simulink library "Cooling"  (R2024a)
settings: Solver=VariableStepAuto  StartTime=0.0  StopTime=10.0  RelTol=1e-3
values from neighbouring files (symbols this model uses):
  VehicleState : value not decoded    [StateMachine.sldd]
undefined symbols (not defined in the file or in its folder): raptor_xcp_function
libraries: $bdroot x11, Raptor_lib x9, simulink x6, Utilities x3
settings Model: Creator=serga  LastModifiedBy=hyuga
settings ConfigComp: CovBoundaryAbsTol=1.0e-5

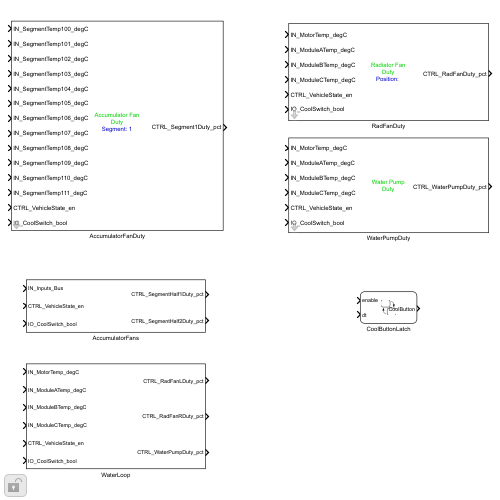
[thumbnail: Simulink's stored preview of the top-level diagram]
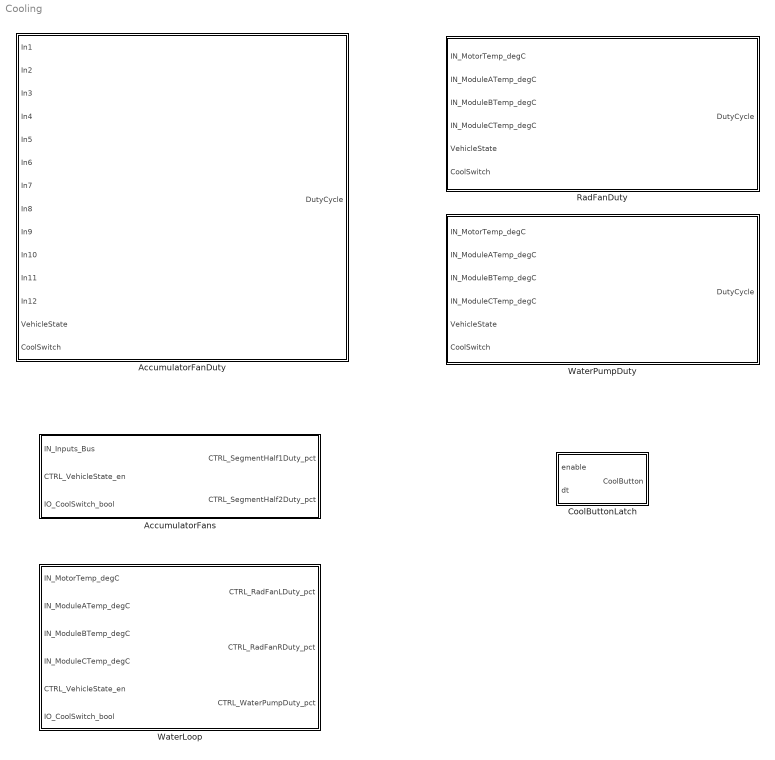
== system Cooling ==
  AccumulatorFanDuty : Subsystem  mask{pos='1'}
      mask prompts: pos "Segment"
      mask Display:
      | color('green')
      | disp('Accumulator Fan\nDuty\n\n');
      | color('blue')
      | disp(['\nSegment: ' pos]);
      | color('black')
      | port_label('input', 1, ['IN_SegmentTemp' pos '00_degC']);
      | port_label('input', 2, ['IN_SegmentTemp' pos '01_degC']);
      | port_label('input', 3, ['IN_SegmentTemp' pos '02_degC']);
      | port_label('input', 4, ['IN_SegmentTemp' pos '03_degC']);
      | port_label('input', 5, ['IN_SegmentTemp' pos '04_degC']);
      | port_label('input', 6, ['IN_SegmentTemp' pos '05_degC']);
      | port_label('input', 7, ['IN_SegmentTemp' pos '06_degC']);
      | port_label('input', 8, ['IN_SegmentTemp' pos '07_degC']);
      | port_label('input', 9, ['IN_SegmentTemp' pos '08_degC']);
      | port_label('input', 10, ['IN_SegmentTemp' pos '09_degC']);
      | port_label('input', 11, ['IN_SegmentTemp' pos '10_degC']);
      | port_label('input', 12, ['IN_SegmentTemp' pos '11_degC']);
      | port_label('input', 13, 'CTRL_VehicleState_en');
      | port_label('input', 14, 'IO_CoolSwitch_bool');
      | port_label('output', 1, ['CTRL_Segment' pos 'Duty_pct']);
  AccumulatorFans : Subsystem
  CoolButtonLatch : Stateflow chart  TreatAsAtomicUnit=on
  RadFanDuty : Subsystem  mask{pos=''}
      mask prompts: pos "Position"
      mask Display:
      | color('green')
      | disp('Radiator Fan\nDuty\n');
      | color('blue')
      | disp(['\n\nPosition: ' pos]);
      | color('black')
      | port_label('input', 1, 'IN_MotorTemp_degC');
      | port_label('input', 2, 'IN_ModuleATemp_degC');
      | port_label('input', 3, 'IN_ModuleBTemp_degC');
      | port_label('input', 4, 'IN_ModuleCTemp_degC');
      | port_label('input', 5, 'CTRL_VehicleState_en');
      | port_label('input', 6, 'IO_CoolSwitch_bool');
      | port_label('output', 1, ['CTRL_RadFan' pos 'Duty_pct']);
  WaterLoop : Subsystem
  WaterPumpDuty : Subsystem
      mask Display:
      | color('green')
      | disp('Water Pump\nDuty');
      | % color('blue')
      | % disp(['\nPosition: ' pos]);
      | color('black')
      | port_label('input', 1, 'IN_MotorTemp_degC');
      | port_label('input', 2, 'IN_ModuleATemp_degC');
      | port_label('input', 3, 'IN_ModuleBTemp_degC');
      | port_label('input', 4, 'IN_ModuleCTemp_degC');
      | port_label('input', 5, 'CTRL_VehicleState_en');
      | port_label('input', 6, 'IO_CoolSwitch_bool');
      | port_label('output', 1, 'CTRL_WaterPumpDuty_pct');

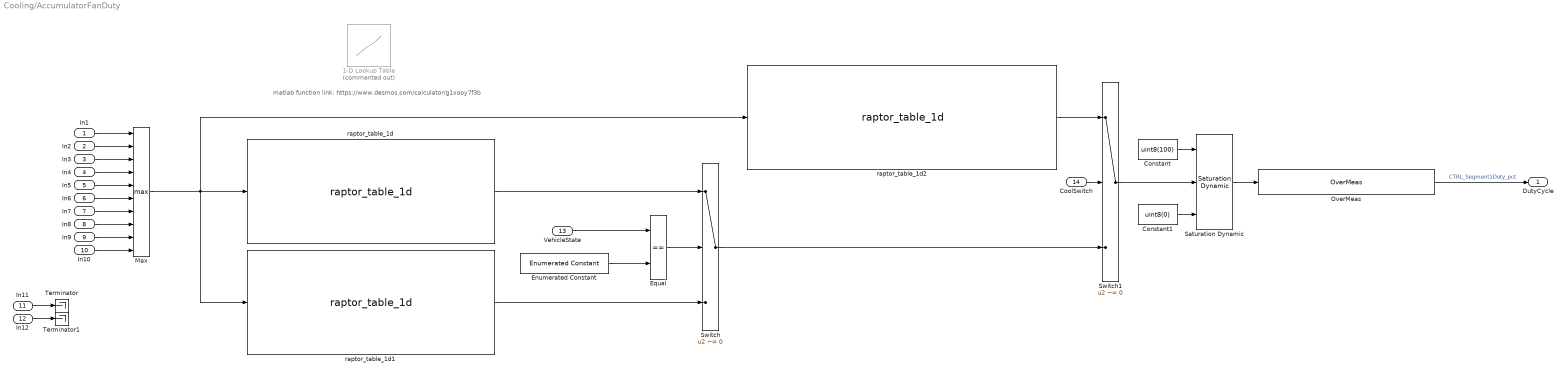
== system Cooling/AccumulatorFanDuty ==
  note: matlab function link: https://www.desmos.com/calculator/g1xooy7f3b
  In1 : Inport
  In2 : Inport  Port=2
  In3 : Inport  Port=3
  In4 : Inport  Port=4
  In5 : Inport  Port=5
  In6 : Inport  Port=6
  In7 : Inport  Port=7
  In8 : Inport  Port=8
  In9 : Inport  Port=9
  In10 : Inport  Port=10
  In11 : Inport  Port=11
  In12 : Inport  Port=12
  VehicleState : Inport  Port=13
  CoolSwitch : Inport  Port=14
  1-D Lookup Table : Lookup_n-D  Commented=on  NumberOfTableDimensions=1  BreakpointsForDimension1=[0:100]  Table=min(((tanh(([0:100]-40)/20)*50+50).^1.03),100)  InternalRulePriority=Speed  RndMeth=Simplest
  Constant : Constant  Value=uint8(100)
  Constant1 : Constant  Value=uint8(0)
  Enumerated Constant : simulink/Sources/Enumerated Constant  OutDataTypeStr=Enum: VehicleState  Value=VehicleState.ReadyToMove  SampleTime=inf
  Equal : RelationalOperator  Operator===  OutDataTypeStr=boolean  RndMeth=Simplest  InputSameDT=off
  Max : MinMax  Function=max  Inputs=10
  OverMeas : Utilities/OverMeas  sigName=['CTRL_Segment' pos 'Duty_pct']  minimum=0  maximum=100
  Saturation Dynamic : simulink/Discontinuities/Saturation Dynamic  OutMin=[]  OutMax=[]  OutDataTypeStr=Inherit: Same as second input  OutDataType=fixdt(1, 16)  OutScaling=2^-10  DoSatur=off
  Switch : Switch  Criteria=u2 ~= 0  SaturateOnIntegerOverflow=off  InputSameDT=off
  Switch1 : Switch  Criteria=u2 ~= 0  SaturateOnIntegerOverflow=off  InputSameDT=off
  Terminator : Terminator
  Terminator1 : Terminator
  raptor_table_1d : Raptor_lib/Table Lookup/raptor_table_1d  dataName=['CTRL_Segment' pos 'TempToHVDutyCycle']  initValue=min(((tanh(([0:100]-40)/20)*50+50).^1.03),80)  dataType=single  storage=Calibration  initValueX=[0:100]  dataTypeXY=single  storageXY=Calibration  calVisible=on  showTable=on  calGain=1.0  calOffset=0.0  calMax=Inf  calMin=-Inf  calFormat='-1'  calUnit='pct'  calHelp=''  showBreakpoint=on  dataNameX=[]  calGainX=1.0  calOffsetX=0.0  calMaxX=Inf  calMinX=-Inf  calFormatX='-1'  calUnitX='degC'  calHelpX=''  calAccess=1  calFunction=raptor_xcp_function(gcb)  measureEnable=off  mName=['Data1D_Output']
      settings: SourceProductName=Raptor
  raptor_table_1d1 : Raptor_lib/Table Lookup/raptor_table_1d  dataName=['CTRL_Segment' pos 'TempToLVDutyCycle']  initValue=min(((tanh(([0:100]-50)/20)*50+50).^1.03),50)  dataType=single  storage=Calibration  initValueX=[0:100]  dataTypeXY=single  storageXY=Calibration  calVisible=on  showTable=on  calGain=1.0  calOffset=0.0  calMax=Inf  calMin=-Inf  calFormat='-1'  calUnit='pct'  calHelp=''  showBreakpoint=on  dataNameX=[]  calGainX=1.0  calOffsetX=0.0  calMaxX=Inf  calMinX=-Inf  calFormatX='-1'  calUnitX='degC'  calHelpX=''  calAccess=1  calFunction=raptor_xcp_function(gcb)  measureEnable=off  mName=['Data1D_Output']
      settings: SourceProductName=Raptor
  raptor_table_1d2 : Raptor_lib/Table Lookup/raptor_table_1d  dataName=['CTRL_Segment' pos 'TempToDutyCycleOverride']  initValue=min(((tanh(([0:100]-25)/20)*50+50).^1.03),100)  dataType=single  storage=Calibration  initValueX=[0:100]  dataTypeXY=single  storageXY=Calibration  calVisible=on  showTable=on  calGain=1.0  calOffset=0.0  calMax=Inf  calMin=-Inf  calFormat='-1'  calUnit='pct'  calHelp=''  showBreakpoint=on  dataNameX=[]  calGainX=1.0  calOffsetX=0.0  calMaxX=Inf  calMinX=-Inf  calFormatX='-1'  calUnitX='degC'  calHelpX=''  calAccess=1  calFunction=raptor_xcp_function(gcb)  measureEnable=off  mName=['Data1D_Output']
      settings: SourceProductName=Raptor
  DutyCycle : Outport
  wires:
  In1/1 -> Max/1
  In2/1 -> Max/2
  In3/1 -> Max/3
  In4/1 -> Max/4
  In5/1 -> Max/5
  In6/1 -> Max/6
  In7/1 -> Max/7
  In8/1 -> Max/8
  In9/1 -> Max/9
  In10/1 -> Max/10
  In11/1 -> Terminator/1
  In12/1 -> Terminator1/1
  Max/1 -> raptor_table_1d1/1, raptor_table_1d2/1, raptor_table_1d/1
  raptor_table_1d/1 -> Switch/1
  VehicleState/1 -> Equal/1
  Enumerated Constant/1 -> Equal/2
  Equal/1 -> Switch/2
  Switch/1 -> Switch1/3
  raptor_table_1d1/1 -> Switch/3
  CoolSwitch/1 -> Switch1/2
  raptor_table_1d2/1 -> Switch1/1
  Switch1/1 -> Saturation Dynamic/2
  Constant/1 -> Saturation Dynamic/1
  Constant1/1 -> Saturation Dynamic/3
  Saturation Dynamic/1 -> OverMeas/1
  OverMeas/1 -> DutyCycle/1  "CTRL_Segment1Duty_pct"

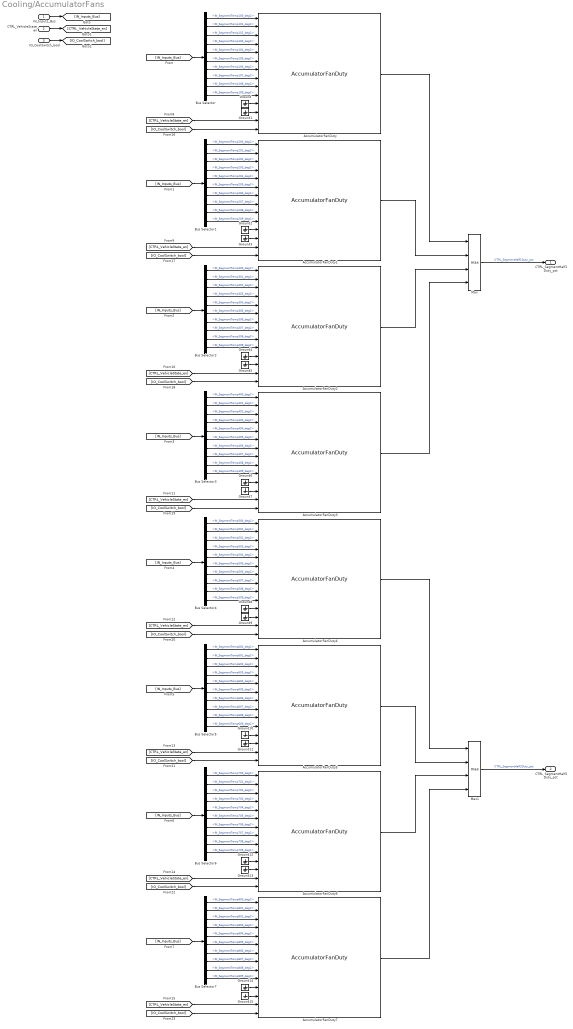
== system Cooling/AccumulatorFans ==
  IN_Inputs_Bus : Inport
  CTRL_VehicleState_en : Inport  Port=2
  IO_CoolSwitch_bool : Inport  Port=3
  AccumulatorFanDuty : $bdroot/AccumulatorFanDuty  pos='1'
  AccumulatorFanDuty1 : $bdroot/AccumulatorFanDuty  pos='2'
  AccumulatorFanDuty2 : $bdroot/AccumulatorFanDuty  pos='3'
  AccumulatorFanDuty3 : $bdroot/AccumulatorFanDuty  pos='4'
  AccumulatorFanDuty4 : $bdroot/AccumulatorFanDuty  pos='5'
  AccumulatorFanDuty5 : $bdroot/AccumulatorFanDuty  pos='6'
  AccumulatorFanDuty6 : $bdroot/AccumulatorFanDuty  pos='7'
  AccumulatorFanDuty7 : $bdroot/AccumulatorFanDuty  pos='8'
  Bus Selector : BusSelector  OutputSignals=IN_STMM_Bus.IN_Segment1Temp_Bus.IN_SegmentTemp100_degC,IN_STMM_Bus.IN_Segment1Temp_Bus.IN_SegmentTemp101_degC,IN_STMM_Bus.IN_Segment1Temp_Bus.IN_SegmentTemp102_degC,IN_STMM_Bus.IN_Segment1Temp_Bus.IN_SegmentTemp103_degC,IN_STMM_Bus.IN_Segment1Temp_Bus.IN_SegmentTemp104_degC,IN_STMM_Bus.IN_Segment1Temp_Bus.IN_SegmentTemp105_degC,IN_STMM_Bus.IN_Segment1Temp_Bus.IN_SegmentTemp106_degC,IN_STMM_Bus.IN_Segment1Temp_Bus.IN_SegmentTemp107_degC,IN_STMM_Bus.IN_Segment1Temp_Bus.IN_SegmentTemp108_degC,IN_STMM_Bus.IN_Segment1Temp_Bus.IN_SegmentTemp109_degC
  Bus Selector1 : BusSelector  OutputSignals=IN_STMM_Bus.IN_Segment2Temp_Bus.IN_SegmentTemp200_degC,IN_STMM_Bus.IN_Segment2Temp_Bus.IN_SegmentTemp201_degC,IN_STMM_Bus.IN_Segment2Temp_Bus.IN_SegmentTemp202_degC,IN_STMM_Bus.IN_Segment2Temp_Bus.IN_SegmentTemp203_degC,IN_STMM_Bus.IN_Segment2Temp_Bus.IN_SegmentTemp204_degC,IN_STMM_Bus.IN_Segment2Temp_Bus.IN_SegmentTemp205_degC,IN_STMM_Bus.IN_Segment2Temp_Bus.IN_SegmentTemp206_degC,IN_STMM_Bus.IN_Segment2Temp_Bus.IN_SegmentTemp207_degC,IN_STMM_Bus.IN_Segment2Temp_Bus.IN_SegmentTemp208_degC,IN_STMM_Bus.IN_Segment2Temp_Bus.IN_SegmentTemp209_degC
  Bus Selector2 : BusSelector  OutputSignals=IN_STMM_Bus.IN_Segment3Temp_Bus.IN_SegmentTemp300_degC,IN_STMM_Bus.IN_Segment3Temp_Bus.IN_SegmentTemp301_degC,IN_STMM_Bus.IN_Segment3Temp_Bus.IN_SegmentTemp302_degC,IN_STMM_Bus.IN_Segment3Temp_Bus.IN_SegmentTemp303_degC,IN_STMM_Bus.IN_Segment3Temp_Bus.IN_SegmentTemp304_degC,IN_STMM_Bus.IN_Segment3Temp_Bus.IN_SegmentTemp305_degC,IN_STMM_Bus.IN_Segment3Temp_Bus.IN_SegmentTemp306_degC,IN_STMM_Bus.IN_Segment3Temp_Bus.IN_SegmentTemp307_degC,IN_STMM_Bus.IN_Segment3Temp_Bus.IN_SegmentTemp308_degC,IN_STMM_Bus.IN_Segment3Temp_Bus.IN_SegmentTemp309_degC
  Bus Selector3 : BusSelector  OutputSignals=IN_STMM_Bus.IN_Segment4Temp_Bus.IN_SegmentTemp400_degC,IN_STMM_Bus.IN_Segment4Temp_Bus.IN_SegmentTemp401_degC,IN_STMM_Bus.IN_Segment4Temp_Bus.IN_SegmentTemp402_degC,IN_STMM_Bus.IN_Segment4Temp_Bus.IN_SegmentTemp403_degC,IN_STMM_Bus.IN_Segment4Temp_Bus.IN_SegmentTemp404_degC,IN_STMM_Bus.IN_Segment4Temp_Bus.IN_SegmentTemp405_degC,IN_STMM_Bus.IN_Segment4Temp_Bus.IN_SegmentTemp406_degC,IN_STMM_Bus.IN_Segment4Temp_Bus.IN_SegmentTemp407_degC,IN_STMM_Bus.IN_Segment4Temp_Bus.IN_SegmentTemp408_degC,IN_STMM_Bus.IN_Segment4Temp_Bus.IN_SegmentTemp409_degC
  Bus Selector4 : BusSelector  OutputSignals=IN_STMM_Bus.IN_Segment5Temp_Bus.IN_SegmentTemp500_degC,IN_STMM_Bus.IN_Segment5Temp_Bus.IN_SegmentTemp501_degC,IN_STMM_Bus.IN_Segment5Temp_Bus.IN_SegmentTemp502_degC,IN_STMM_Bus.IN_Segment5Temp_Bus.IN_SegmentTemp503_degC,IN_STMM_Bus.IN_Segment5Temp_Bus.IN_SegmentTemp504_degC,IN_STMM_Bus.IN_Segment5Temp_Bus.IN_SegmentTemp505_degC,IN_STMM_Bus.IN_Segment5Temp_Bus.IN_SegmentTemp506_degC,IN_STMM_Bus.IN_Segment5Temp_Bus.IN_SegmentTemp507_degC,IN_STMM_Bus.IN_Segment5Temp_Bus.IN_SegmentTemp508_degC,IN_STMM_Bus.IN_Segment5Temp_Bus.IN_SegmentTemp509_degC
  Bus Selector5 : BusSelector  OutputSignals=IN_STMM_Bus.IN_Segment6Temp_Bus.IN_SegmentTemp600_degC,IN_STMM_Bus.IN_Segment6Temp_Bus.IN_SegmentTemp601_degC,IN_STMM_Bus.IN_Segment6Temp_Bus.IN_SegmentTemp602_degC,IN_STMM_Bus.IN_Segment6Temp_Bus.IN_SegmentTemp603_degC,IN_STMM_Bus.IN_Segment6Temp_Bus.IN_SegmentTemp604_degC,IN_STMM_Bus.IN_Segment6Temp_Bus.IN_SegmentTemp605_degC,IN_STMM_Bus.IN_Segment6Temp_Bus.IN_SegmentTemp606_degC,IN_STMM_Bus.IN_Segment6Temp_Bus.IN_SegmentTemp607_degC,IN_STMM_Bus.IN_Segment6Temp_Bus.IN_SegmentTemp608_degC,IN_STMM_Bus.IN_Segment6Temp_Bus.IN_SegmentTemp609_degC
  Bus Selector6 : BusSelector  OutputSignals=IN_STMM_Bus.IN_Segment7Temp_Bus.IN_SegmentTemp700_degC,IN_STMM_Bus.IN_Segment7Temp_Bus.IN_SegmentTemp701_degC,IN_STMM_Bus.IN_Segment7Temp_Bus.IN_SegmentTemp702_degC,IN_STMM_Bus.IN_Segment7Temp_Bus.IN_SegmentTemp703_degC,IN_STMM_Bus.IN_Segment7Temp_Bus.IN_SegmentTemp704_degC,IN_STMM_Bus.IN_Segment7Temp_Bus.IN_SegmentTemp705_degC,IN_STMM_Bus.IN_Segment7Temp_Bus.IN_SegmentTemp706_degC,IN_STMM_Bus.IN_Segment7Temp_Bus.IN_SegmentTemp707_degC,IN_STMM_Bus.IN_Segment7Temp_Bus.IN_SegmentTemp708_degC,IN_STMM_Bus.IN_Segment7Temp_Bus.IN_SegmentTemp709_degC
  Bus Selector7 : BusSelector  OutputSignals=IN_STMM_Bus.IN_Segment8Temp_Bus.IN_SegmentTemp800_degC,IN_STMM_Bus.IN_Segment8Temp_Bus.IN_SegmentTemp801_degC,IN_STMM_Bus.IN_Segment8Temp_Bus.IN_SegmentTemp802_degC,IN_STMM_Bus.IN_Segment8Temp_Bus.IN_SegmentTemp803_degC,IN_STMM_Bus.IN_Segment8Temp_Bus.IN_SegmentTemp804_degC,IN_STMM_Bus.IN_Segment8Temp_Bus.IN_SegmentTemp805_degC,IN_STMM_Bus.IN_Segment8Temp_Bus.IN_SegmentTemp806_degC,IN_STMM_Bus.IN_Segment8Temp_Bus.IN_SegmentTemp807_degC,IN_STMM_Bus.IN_Segment8Temp_Bus.IN_SegmentTemp808_degC,IN_STMM_Bus.IN_Segment8Temp_Bus.IN_SegmentTemp809_degC
  Ground{,1..15} (16 alike) : Ground
  Max : MinMax  Function=max  Inputs=4
  Max1 : MinMax  Function=max  Inputs=4
  CTRL_SegmentHalf1Duty_pct : Outport
  CTRL_SegmentHalf2Duty_pct : Outport  Port=2
  wires:
  Max1/1 -> CTRL_SegmentHalf2Duty_pct/1  "CTRL_SegmentHalf2Duty_pct"
  AccumulatorFanDuty7/1 -> Max1/4
  AccumulatorFanDuty6/1 -> Max1/3
  AccumulatorFanDuty5/1 -> Max1/2
  AccumulatorFanDuty4/1 -> Max1/1
  Max/1 -> CTRL_SegmentHalf1Duty_pct/1  "CTRL_SegmentHalf1Duty_pct"
  AccumulatorFanDuty3/1 -> Max/4
  AccumulatorFanDuty2/1 -> Max/3
  AccumulatorFanDuty1/1 -> Max/2
  AccumulatorFanDuty/1 -> Max/1
  [IO_CoolSwitch_bool] -> AccumulatorFanDuty7/14
  [IO_CoolSwitch_bool] -> AccumulatorFanDuty6/14
  [IO_CoolSwitch_bool] -> AccumulatorFanDuty5/14
  [IO_CoolSwitch_bool] -> AccumulatorFanDuty4/14
  [IO_CoolSwitch_bool] -> AccumulatorFanDuty3/14
  [IO_CoolSwitch_bool] -> AccumulatorFanDuty2/14
  [IO_CoolSwitch_bool] -> AccumulatorFanDuty1/14
  [IO_CoolSwitch_bool] -> AccumulatorFanDuty/14
  [CTRL_VehicleState_en] -> AccumulatorFanDuty7/13
  [CTRL_VehicleState_en] -> AccumulatorFanDuty6/13
  [CTRL_VehicleState_en] -> AccumulatorFanDuty5/13
  [CTRL_VehicleState_en] -> AccumulatorFanDuty4/13
  [CTRL_VehicleState_en] -> AccumulatorFanDuty3/13
  [CTRL_VehicleState_en] -> AccumulatorFanDuty2/13
  [CTRL_VehicleState_en] -> AccumulatorFanDuty1/13
  [CTRL_VehicleState_en] -> AccumulatorFanDuty/13
  [IN_Inputs_Bus] -> Bus Selector7/1
  [IN_Inputs_Bus] -> Bus Selector6/1
  [IN_Inputs_Bus] -> Bus Selector5/1
  [IN_Inputs_Bus] -> Bus Selector4/1
  [IN_Inputs_Bus] -> Bus Selector3/1
  [IN_Inputs_Bus] -> Bus Selector2/1
  [IN_Inputs_Bus] -> Bus Selector1/1
  [IN_Inputs_Bus] -> Bus Selector/1
  IO_CoolSwitch_bool/1 -> [IO_CoolSwitch_bool]
  CTRL_VehicleState_en/1 -> [CTRL_VehicleState_en]
  IN_Inputs_Bus/1 -> [IN_Inputs_Bus]
  Bus Selector7/10 -> AccumulatorFanDuty7/10  "<IN_SegmentTemp809_degC>"
  Bus Selector7/9 -> AccumulatorFanDuty7/9  "<IN_SegmentTemp808_degC>"
  Bus Selector7/8 -> AccumulatorFanDuty7/8  "<IN_SegmentTemp807_degC>"
  Bus Selector7/7 -> AccumulatorFanDuty7/7  "<IN_SegmentTemp806_degC>"
  Bus Selector7/6 -> AccumulatorFanDuty7/6  "<IN_SegmentTemp805_degC>"
  Bus Selector7/5 -> AccumulatorFanDuty7/5  "<IN_SegmentTemp804_degC>"
  Bus Selector7/4 -> AccumulatorFanDuty7/4  "<IN_SegmentTemp803_degC>"
  Bus Selector7/3 -> AccumulatorFanDuty7/3  "<IN_SegmentTemp802_degC>"
  Bus Selector7/2 -> AccumulatorFanDuty7/2  "<IN_SegmentTemp801_degC>"
  Bus Selector7/1 -> AccumulatorFanDuty7/1  "<IN_SegmentTemp800_degC>"
  Bus Selector6/10 -> AccumulatorFanDuty6/10  "<IN_SegmentTemp709_degC>"
  Bus Selector6/9 -> AccumulatorFanDuty6/9  "<IN_SegmentTemp708_degC>"
  Bus Selector6/8 -> AccumulatorFanDuty6/8  "<IN_SegmentTemp707_degC>"
  Bus Selector6/7 -> AccumulatorFanDuty6/7  "<IN_SegmentTemp706_degC>"
  Bus Selector6/6 -> AccumulatorFanDuty6/6  "<IN_SegmentTemp705_degC>"
  Bus Selector6/5 -> AccumulatorFanDuty6/5  "<IN_SegmentTemp704_degC>"
  Bus Selector6/4 -> AccumulatorFanDuty6/4  "<IN_SegmentTemp703_degC>"
  Bus Selector6/3 -> AccumulatorFanDuty6/3  "<IN_SegmentTemp702_degC>"
  Bus Selector6/2 -> AccumulatorFanDuty6/2  "<IN_SegmentTemp701_degC>"
  Bus Selector6/1 -> AccumulatorFanDuty6/1  "<IN_SegmentTemp700_degC>"
  Bus Selector5/10 -> AccumulatorFanDuty5/10  "<IN_SegmentTemp609_degC>"
  Bus Selector5/9 -> AccumulatorFanDuty5/9  "<IN_SegmentTemp608_degC>"
  Bus Selector5/8 -> AccumulatorFanDuty5/8  "<IN_SegmentTemp607_degC>"
  Bus Selector5/7 -> AccumulatorFanDuty5/7  "<IN_SegmentTemp606_degC>"
  Bus Selector5/6 -> AccumulatorFanDuty5/6  "<IN_SegmentTemp605_degC>"
  Bus Selector5/5 -> AccumulatorFanDuty5/5  "<IN_SegmentTemp604_degC>"
  Bus Selector5/4 -> AccumulatorFanDuty5/4  "<IN_SegmentTemp603_degC>"
  Bus Selector5/3 -> AccumulatorFanDuty5/3  "<IN_SegmentTemp602_degC>"
  Bus Selector5/2 -> AccumulatorFanDuty5/2  "<IN_SegmentTemp601_degC>"
  Bus Selector5/1 -> AccumulatorFanDuty5/1  "<IN_SegmentTemp600_degC>"
  Bus Selector4/10 -> AccumulatorFanDuty4/10  "<IN_SegmentTemp509_degC>"
  Bus Selector4/9 -> AccumulatorFanDuty4/9  "<IN_SegmentTemp508_degC>"
  Bus Selector4/8 -> AccumulatorFanDuty4/8  "<IN_SegmentTemp507_degC>"
  Bus Selector4/7 -> AccumulatorFanDuty4/7  "<IN_SegmentTemp506_degC>"
  Bus Selector4/6 -> AccumulatorFanDuty4/6  "<IN_SegmentTemp505_degC>"
  Bus Selector4/5 -> AccumulatorFanDuty4/5  "<IN_SegmentTemp504_degC>"
  Bus Selector4/4 -> AccumulatorFanDuty4/4  "<IN_SegmentTemp503_degC>"
  Bus Selector4/3 -> AccumulatorFanDuty4/3  "<IN_SegmentTemp502_degC>"
  Bus Selector4/2 -> AccumulatorFanDuty4/2  "<IN_SegmentTemp501_degC>"
  Bus Selector4/1 -> AccumulatorFanDuty4/1  "<IN_SegmentTemp500_degC>"
  Bus Selector3/10 -> AccumulatorFanDuty3/10  "<IN_SegmentTemp409_degC>"
  Bus Selector3/9 -> AccumulatorFanDuty3/9  "<IN_SegmentTemp408_degC>"
  Bus Selector3/8 -> AccumulatorFanDuty3/8  "<IN_SegmentTemp407_degC>"
  Bus Selector3/7 -> AccumulatorFanDuty3/7  "<IN_SegmentTemp406_degC>"
  Bus Selector3/6 -> AccumulatorFanDuty3/6  "<IN_SegmentTemp405_degC>"
  Bus Selector3/5 -> AccumulatorFanDuty3/5  "<IN_SegmentTemp404_degC>"
  Bus Selector3/4 -> AccumulatorFanDuty3/4  "<IN_SegmentTemp403_degC>"
  Bus Selector3/3 -> AccumulatorFanDuty3/3  "<IN_SegmentTemp402_degC>"
  Bus Selector3/2 -> AccumulatorFanDuty3/2  "<IN_SegmentTemp401_degC>"
  Bus Selector3/1 -> AccumulatorFanDuty3/1  "<IN_SegmentTemp400_degC>"
  Bus Selector2/10 -> AccumulatorFanDuty2/10  "<IN_SegmentTemp309_degC>"
  Bus Selector2/9 -> AccumulatorFanDuty2/9  "<IN_SegmentTemp308_degC>"
  Bus Selector2/8 -> AccumulatorFanDuty2/8  "<IN_SegmentTemp307_degC>"
  Bus Selector2/7 -> AccumulatorFanDuty2/7  "<IN_SegmentTemp306_degC>"
  Bus Selector2/6 -> AccumulatorFanDuty2/6  "<IN_SegmentTemp305_degC>"
  Bus Selector2/5 -> AccumulatorFanDuty2/5  "<IN_SegmentTemp304_degC>"
  Bus Selector2/4 -> AccumulatorFanDuty2/4  "<IN_SegmentTemp303_degC>"
  Bus Selector2/3 -> AccumulatorFanDuty2/3  "<IN_SegmentTemp302_degC>"
  Bus Selector2/2 -> AccumulatorFanDuty2/2  "<IN_SegmentTemp301_degC>"
  Bus Selector2/1 -> AccumulatorFanDuty2/1  "<IN_SegmentTemp300_degC>"
  Bus Selector1/10 -> AccumulatorFanDuty1/10  "<IN_SegmentTemp209_degC>"
  Bus Selector1/9 -> AccumulatorFanDuty1/9  "<IN_SegmentTemp208_degC>"
  Bus Selector1/8 -> AccumulatorFanDuty1/8  "<IN_SegmentTemp207_degC>"
  Bus Selector1/7 -> AccumulatorFanDuty1/7  "<IN_SegmentTemp206_degC>"
  Bus Selector1/6 -> AccumulatorFanDuty1/6  "<IN_SegmentTemp205_degC>"
  Bus Selector1/5 -> AccumulatorFanDuty1/5  "<IN_SegmentTemp204_degC>"
  Bus Selector1/4 -> AccumulatorFanDuty1/4  "<IN_SegmentTemp203_degC>"
  Bus Selector1/3 -> AccumulatorFanDuty1/3  "<IN_SegmentTemp202_degC>"
  Bus Selector1/2 -> AccumulatorFanDuty1/2  "<IN_SegmentTemp201_degC>"
  Bus Selector1/1 -> AccumulatorFanDuty1/1  "<IN_SegmentTemp200_degC>"
  Bus Selector/10 -> AccumulatorFanDuty/10  "<IN_SegmentTemp109_degC>"
  Bus Selector/9 -> AccumulatorFanDuty/9  "<IN_SegmentTemp108_degC>"
  Bus Selector/8 -> AccumulatorFanDuty/8  "<IN_SegmentTemp107_degC>"
  Bus Selector/7 -> AccumulatorFanDuty/7  "<IN_SegmentTemp106_degC>"
  Bus Selector/6 -> AccumulatorFanDuty/6  "<IN_SegmentTemp105_degC>"
  Bus Selector/5 -> AccumulatorFanDuty/5  "<IN_SegmentTemp104_degC>"
  Bus Selector/4 -> AccumulatorFanDuty/4  "<IN_SegmentTemp103_degC>"
  Bus Selector/3 -> AccumulatorFanDuty/3  "<IN_SegmentTemp102_degC>"
  Bus Selector/2 -> AccumulatorFanDuty/2  "<IN_SegmentTemp101_degC>"
  Bus Selector/1 -> AccumulatorFanDuty/1  "<IN_SegmentTemp100_degC>"
  Ground/1 -> AccumulatorFanDuty/11
  Ground1/1 -> AccumulatorFanDuty/12
  Ground2/1 -> AccumulatorFanDuty1/11
  Ground3/1 -> AccumulatorFanDuty1/12
  Ground4/1 -> AccumulatorFanDuty2/11
  Ground5/1 -> AccumulatorFanDuty2/12
  Ground6/1 -> AccumulatorFanDuty3/11
  Ground7/1 -> AccumulatorFanDuty3/12
  Ground8/1 -> AccumulatorFanDuty4/11
  Ground9/1 -> AccumulatorFanDuty4/12
  Ground10/1 -> AccumulatorFanDuty5/11
  Ground11/1 -> AccumulatorFanDuty5/12
  Ground12/1 -> AccumulatorFanDuty6/11
  Ground13/1 -> AccumulatorFanDuty6/12
  Ground14/1 -> AccumulatorFanDuty7/11
  Ground15/1 -> AccumulatorFanDuty7/12

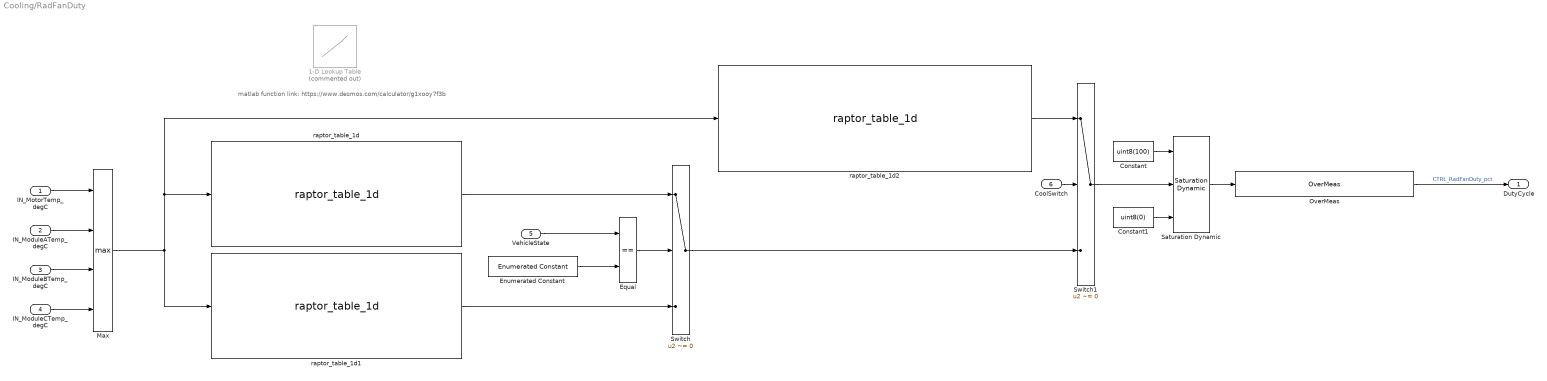
== system Cooling/RadFanDuty ==
  note: matlab function link: https://www.desmos.com/calculator/g1xooy7f3b
  IN_MotorTemp_degC : Inport
  IN_ModuleATemp_degC : Inport  Port=2
  IN_ModuleBTemp_degC : Inport  Port=3
  IN_ModuleCTemp_degC : Inport  Port=4
  VehicleState : Inport  Port=5
  CoolSwitch : Inport  Port=6
  1-D Lookup Table : Lookup_n-D  Commented=on  NumberOfTableDimensions=1  BreakpointsForDimension1=[0; 1; 2; 3; 4; 5; 6; 7; 8; 9; 10; 11; 12; 13; 14; 15; 16; 17; 18; 19; 20; 21; 22; 23; 24; 25; 26; 27; 28; 29; 30; 31; 32; 33; 34; 35; 36; 37; 38; 39; 40; 41; 42; 43; 44; 45; 46; 47; 48; 49; 50; 51; 52; 53; 54; 55; 56; 57; 58; 59; 60; 61; 62; 63; 64; 65; 66; 67; 68; 69; 70; 71; 72; 73; 74; 75; 76; 77; 78; 79; 80; 81; 82; 83; 84; 85; 86; 87; 88; 89; 90; 91; 92; 93; 94; 95; 96; 97; 98; 99; 100; 101; 102; 103; 104; 105; 106; 107; 108; 109; 110; 111; 112; 113; 114; 115; 116; 117; 118]  Table=[2, 2, 2, 2, 3, 3, 3, 4, 4, 5, 5, 5, 6, 7, 7, 8, 9, 10, 11, 12, 13, 14, 15, 17, 18, 20, 22, 23, 25, 28, 30, 32, 34, 37, 39, 42, 45, 48, 50, 53, 56, 59, 62, 65, 68, 70, 73, 76, 78, 81, 83, 85, 88, 90, 91, 93, 95, 97, 98, 99, 100, 100, 100, 100, 100, 100, 100, 100, 100, 100, 100, 100, 100, 100, 100, 100, 100, 100, 100, 100, 100, 100, 100, 100, 100, 100, 100, 100, 100, 100, 100, 100, 100, 100, 100, 100, 100, 100, 100, 100, 100, 100, 100, 100, 100, 100, 100, 100, 100, 100, 100, 100, 100, 100, 100, 100, 100, 100, 100]  InternalRulePriority=Speed  RndMeth=Simplest
  Constant : Constant  Value=uint8(100)
  Constant1 : Constant  Value=uint8(0)
  Enumerated Constant : simulink/Sources/Enumerated Constant  OutDataTypeStr=Enum: VehicleState  Value=VehicleState.ReadyToMove  SampleTime=inf
  Equal : RelationalOperator  Operator===  OutDataTypeStr=boolean  RndMeth=Simplest  InputSameDT=off
  Max : MinMax  Function=max  Inputs=4
  OverMeas : Utilities/OverMeas  sigName=['CTRL_RadFan' pos 'Duty_pct']  minimum=0  maximum=100
  Saturation Dynamic : simulink/Discontinuities/Saturation Dynamic  OutMin=[]  OutMax=[]  OutDataTypeStr=Inherit: Same as second input  OutDataType=fixdt(1, 16)  OutScaling=2^-10  DoSatur=off
  Switch : Switch  Criteria=u2 ~= 0  SaturateOnIntegerOverflow=off  InputSameDT=off
  Switch1 : Switch  Criteria=u2 ~= 0  SaturateOnIntegerOverflow=off  InputSameDT=off
  raptor_table_1d : Raptor_lib/Table Lookup/raptor_table_1d  dataName=['CTRL_RadFan' pos 'TempToHVDutyCycle']  initValue=[0, 0, 0, 0, 0, 0, 0, 0, 0, 0, 0, 0, 0, 0, 0, 0, 0, 0, 0, 0, 0, 0, 0, 0, 0, 0, 0, 0, 0, 0, 0, 0, 0, 0, 0, 0, 0, 0, 0, 0, 0, 0, 0, 0, 0, 0, 0, 0, 0, 0, 0, 0, 0, 0, 0, 0, 0, 0, 0, 0, 0, 0, 0, 0, 0, 0, 100, 100, 100, 100, 100, 100, 100, 100, 100, 100, 100, 100, 100, 100, 100, 100, 100, 100, 100, 100, 100, 100, 100, 100, 100, 100, 100, 100, 100, 100, 100, 100, 100, 100, 100, 100, 100, 100, 100, 100, 100, 100, 100, 100, 100, 100, 100, 100, 100, 100, 100, 100, 100]  dataType=single  storage=Calibration  initValueX=[0; 1; 2; 3; 4; 5; 6; 7; 8; 9; 10; 11; 12; 13; 14; 15; 16; 17; 18; 19; 20; 21; 22; 23; 24; 25; 26; 27; 28; 29; 30; 31; 32; 33; 34; 35; 36; 37; 38; 39; 40; 41; 42; 43; 44; 45; 46; 47; 48; 49; 50; 51; 52; 53; 54; 55; 56; 57; 58; 59; 60; 61; 62; 63; 64; 65; 66; 67; 68; 69; 70; 71; 72; 73; 74; 75; 76; 77; 78; 79; 80; 81; 82; 83; 84; 85; 86; 87; 88; 89; 90; 91; 92; 93; 94; 95; 96; 97; 98; 99; 100; 101; 102; 103; 104; 105; 106; 107; 108; 109; 110; 111; 112; 113; 114; 115; 116; 117; 118]  dataTypeXY=single  storageXY=Calibration  calVisible=on  showTable=on  calGain=1.0  calOffset=0.0  calMax=Inf  calMin=-Inf  calFormat='-1'  calUnit='pct'  calHelp=''  showBreakpoint=on  dataNameX=[]  calGainX=1.0  calOffsetX=0.0  calMaxX=Inf  calMinX=-Inf  calFormatX='-1'  calUnitX='degC'  calHelpX=''  calAccess=1  calFunction=raptor_xcp_function(gcb)  measureEnable=off  mName=['Data1D_Output']
      settings: SourceProductName=Raptor
  raptor_table_1d1 : Raptor_lib/Table Lookup/raptor_table_1d  dataName=['CTRL_RadFan' pos 'TempToLVDutyCycle']  initValue=[0, 0, 0, 0, 0, 0, 0, 0, 0, 0, 0, 0, 0, 0, 0, 0, 0, 0, 0, 0, 0, 0, 0, 0, 0, 0, 0, 0, 0, 0, 0, 0, 0, 0, 0, 0, 0, 0, 0, 0, 0, 0, 0, 0, 0, 0, 0, 0, 0, 0, 0, 0, 0, 0, 0, 0, 0, 0, 0, 0, 0, 0, 0, 0, 0, 0, 100, 100, 100, 100, 100, 100, 100, 100, 100, 100, 100, 100, 100, 100, 100, 100, 100, 100, 100, 100, 100, 100, 100, 100, 100, 100, 100, 100, 100, 100, 100, 100, 100, 100, 100, 100, 100, 100, 100, 100, 100, 100, 100, 100, 100, 100, 100, 100, 100, 100, 100, 100, 100]  dataType=single  storage=Calibration  initValueX=[0; 1; 2; 3; 4; 5; 6; 7; 8; 9; 10; 11; 12; 13; 14; 15; 16; 17; 18; 19; 20; 21; 22; 23; 24; 25; 26; 27; 28; 29; 30; 31; 32; 33; 34; 35; 36; 37; 38; 39; 40; 41; 42; 43; 44; 45; 46; 47; 48; 49; 50; 51; 52; 53; 54; 55; 56; 57; 58; 59; 60; 61; 62; 63; 64; 65; 66; 67; 68; 69; 70; 71; 72; 73; 74; 75; 76; 77; 78; 79; 80; 81; 82; 83; 84; 85; 86; 87; 88; 89; 90; 91; 92; 93; 94; 95; 96; 97; 98; 99; 100; 101; 102; 103; 104; 105; 106; 107; 108; 109; 110; 111; 112; 113; 114; 115; 116; 117; 118]  dataTypeXY=single  storageXY=Calibration  calVisible=on  showTable=on  calGain=1.0  calOffset=0.0  calMax=Inf  calMin=-Inf  calFormat='-1'  calUnit='pct'  calHelp=''  showBreakpoint=on  dataNameX=[]  calGainX=1.0  calOffsetX=0.0  calMaxX=Inf  calMinX=-Inf  calFormatX='-1'  calUnitX='degC'  calHelpX=''  calAccess=1  calFunction=raptor_xcp_function(gcb)  measureEnable=off  mName=['Data1D_Output']
      settings: SourceProductName=Raptor
  raptor_table_1d2 : Raptor_lib/Table Lookup/raptor_table_1d  dataName=['CTRL_RadFan' pos 'TempToDutyCycleOverride']  initValue=[0, 0, 0, 0, 0, 0, 0, 0, 0, 0, 0, 0, 0, 0, 0, 0, 0, 0, 0, 0, 0, 0, 0, 0, 0, 0, 0, 0, 0, 0, 0, 0, 0, 0, 0, 0, 0, 0, 0, 0, 0, 0, 0, 0, 0, 0, 0, 0, 0, 0, 0, 0, 0, 0, 0, 0, 0, 0, 0, 0, 0, 0, 0, 0, 0, 0, 100, 100, 100, 100, 100, 100, 100, 100, 100, 100, 100, 100, 100, 100, 100, 100, 100, 100, 100, 100, 100, 100, 100, 100, 100, 100, 100, 100, 100, 100, 100, 100, 100, 100, 100, 100, 100, 100, 100, 100, 100, 100, 100, 100, 100, 100, 100, 100, 100, 100, 100, 100, 100]  dataType=single  storage=Calibration  initValueX=[0; 1; 2; 3; 4; 5; 6; 7; 8; 9; 10; 11; 12; 13; 14; 15; 16; 17; 18; 19; 20; 21; 22; 23; 24; 25; 26; 27; 28; 29; 30; 31; 32; 33; 34; 35; 36; 37; 38; 39; 40; 41; 42; 43; 44; 45; 46; 47; 48; 49; 50; 51; 52; 53; 54; 55; 56; 57; 58; 59; 60; 61; 62; 63; 64; 65; 66; 67; 68; 69; 70; 71; 72; 73; 74; 75; 76; 77; 78; 79; 80; 81; 82; 83; 84; 85; 86; 87; 88; 89; 90; 91; 92; 93; 94; 95; 96; 97; 98; 99; 100; 101; 102; 103; 104; 105; 106; 107; 108; 109; 110; 111; 112; 113; 114; 115; 116; 117; 118]  dataTypeXY=single  storageXY=Calibration  calVisible=on  showTable=on  calGain=1.0  calOffset=0.0  calMax=Inf  calMin=-Inf  calFormat='-1'  calUnit='pct'  calHelp=''  showBreakpoint=on  dataNameX=[]  calGainX=1.0  calOffsetX=0.0  calMaxX=Inf  calMinX=-Inf  calFormatX='-1'  calUnitX='degC'  calHelpX=''  calAccess=1  calFunction=raptor_xcp_function(gcb)  measureEnable=off  mName=['Data1D_Output']
      settings: SourceProductName=Raptor
  DutyCycle : Outport
  wires:
  IN_MotorTemp_degC/1 -> Max/1
  Equal/1 -> Switch/2
  OverMeas/1 -> DutyCycle/1  "CTRL_RadFanDuty_pct"
  Constant1/1 -> Saturation Dynamic/3
  raptor_table_1d1/1 -> Switch/3
  Saturation Dynamic/1 -> OverMeas/1
  Max/1 -> raptor_table_1d1/1, raptor_table_1d2/1, raptor_table_1d/1
  Constant/1 -> Saturation Dynamic/1
  raptor_table_1d2/1 -> Switch1/1
  Switch1/1 -> Saturation Dynamic/2
  Switch/1 -> Switch1/3
  CoolSwitch/1 -> Switch1/2
  Enumerated Constant/1 -> Equal/2
  VehicleState/1 -> Equal/1
  raptor_table_1d/1 -> Switch/1
  IN_ModuleCTemp_degC/1 -> Max/4
  IN_ModuleBTemp_degC/1 -> Max/3
  IN_ModuleATemp_degC/1 -> Max/2

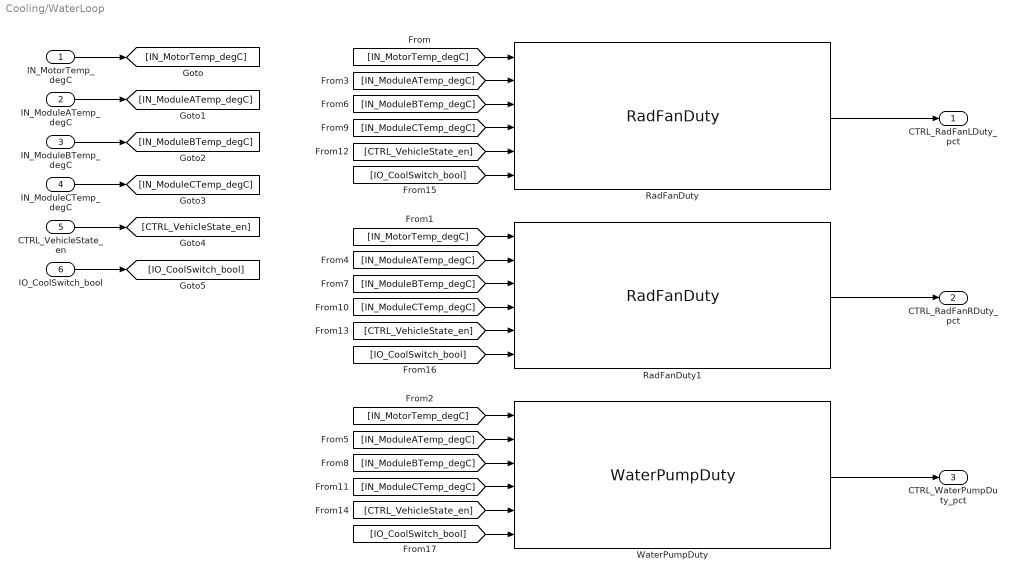
== system Cooling/WaterLoop ==
  IN_MotorTemp_degC : Inport
  IN_ModuleATemp_degC : Inport  Port=2
  IN_ModuleBTemp_degC : Inport  Port=3
  IN_ModuleCTemp_degC : Inport  Port=4
  CTRL_VehicleState_en : Inport  Port=5
  IO_CoolSwitch_bool : Inport  Port=6
  RadFanDuty : $bdroot/RadFanDuty  pos='L'
  RadFanDuty1 : $bdroot/RadFanDuty  pos='R'
  WaterPumpDuty : $bdroot/WaterPumpDuty
  CTRL_RadFanLDuty_pct : Outport
  CTRL_RadFanRDuty_pct : Outport  Port=2
  CTRL_WaterPumpDuty_pct : Outport  Port=3
  wires:
  IN_MotorTemp_degC/1 -> [IN_MotorTemp_degC]
  IN_ModuleATemp_degC/1 -> [IN_ModuleATemp_degC]
  IN_ModuleBTemp_degC/1 -> [IN_ModuleBTemp_degC]
  IN_ModuleCTemp_degC/1 -> [IN_ModuleCTemp_degC]
  CTRL_VehicleState_en/1 -> [CTRL_VehicleState_en]
  IO_CoolSwitch_bool/1 -> [IO_CoolSwitch_bool]
  [IN_MotorTemp_degC] -> RadFanDuty/1
  [IN_MotorTemp_degC] -> RadFanDuty1/1
  [IN_MotorTemp_degC] -> WaterPumpDuty/1
  [IN_ModuleATemp_degC] -> RadFanDuty/2
  [IN_ModuleATemp_degC] -> RadFanDuty1/2
  [IN_ModuleATemp_degC] -> WaterPumpDuty/2
  [IN_ModuleBTemp_degC] -> RadFanDuty/3
  [IN_ModuleBTemp_degC] -> RadFanDuty1/3
  [IN_ModuleBTemp_degC] -> WaterPumpDuty/3
  [IN_ModuleCTemp_degC] -> RadFanDuty/4
  [IN_ModuleCTemp_degC] -> RadFanDuty1/4
  [IN_ModuleCTemp_degC] -> WaterPumpDuty/4
  [CTRL_VehicleState_en] -> RadFanDuty/5
  [CTRL_VehicleState_en] -> RadFanDuty1/5
  [CTRL_VehicleState_en] -> WaterPumpDuty/5
  [IO_CoolSwitch_bool] -> RadFanDuty/6
  [IO_CoolSwitch_bool] -> RadFanDuty1/6
  [IO_CoolSwitch_bool] -> WaterPumpDuty/6
  RadFanDuty/1 -> CTRL_RadFanLDuty_pct/1
  RadFanDuty1/1 -> CTRL_RadFanRDuty_pct/1
  WaterPumpDuty/1 -> CTRL_WaterPumpDuty_pct/1

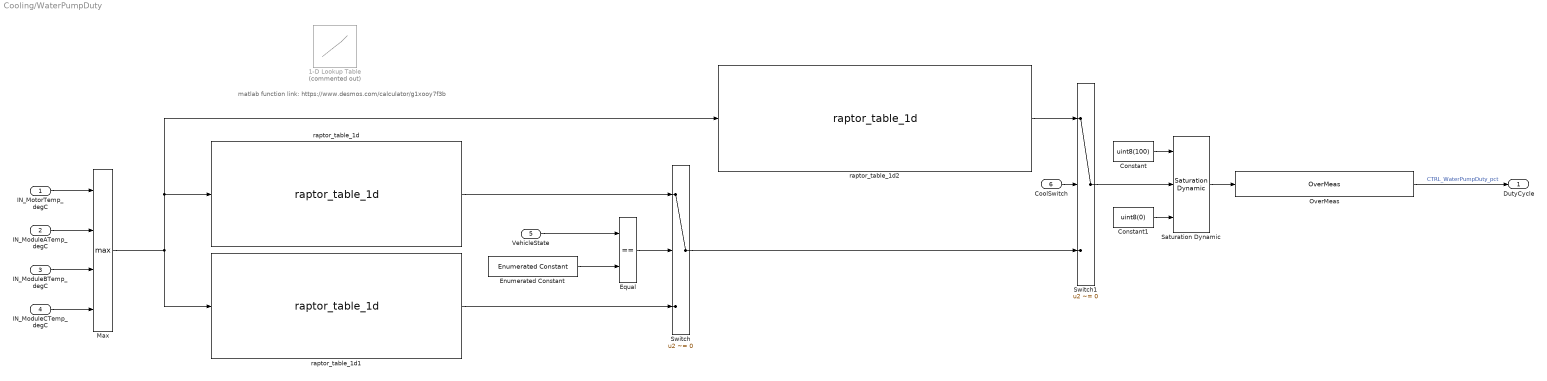
== system Cooling/WaterPumpDuty ==
  note: matlab function link: https://www.desmos.com/calculator/g1xooy7f3b
  IN_MotorTemp_degC : Inport
  IN_ModuleATemp_degC : Inport  Port=2
  IN_ModuleBTemp_degC : Inport  Port=3
  IN_ModuleCTemp_degC : Inport  Port=4
  VehicleState : Inport  Port=5
  CoolSwitch : Inport  Port=6
  1-D Lookup Table : Lookup_n-D  Commented=on  NumberOfTableDimensions=1  BreakpointsForDimension1=[0; 1; 2; 3; 4; 5; 6; 7; 8; 9; 10; 11; 12; 13; 14; 15; 16; 17; 18; 19; 20; 21; 22; 23; 24; 25; 26; 27; 28; 29; 30; 31; 32; 33; 34; 35; 36; 37; 38; 39; 40; 41; 42; 43; 44; 45; 46; 47; 48; 49; 50; 51; 52; 53; 54; 55; 56; 57; 58; 59; 60; 61; 62; 63; 64; 65; 66; 67; 68; 69; 70; 71; 72; 73; 74; 75; 76; 77; 78; 79; 80; 81; 82; 83; 84; 85; 86; 87; 88; 89; 90; 91; 92; 93; 94; 95; 96; 97; 98; 99; 100; 101; 102; 103; 104; 105; 106; 107; 108; 109; 110; 111; 112; 113; 114; 115; 116; 117; 118]  Table=[20, 20, 20, 20, 20, 20, 20, 20, 20, 20, 20, 20, 20, 20, 20, 20, 20, 20, 20, 20, 20, 20, 20, 20, 20, 20, 20, 20, 20, 20, 20, 20, 20, 20, 20, 20, 20, 20, 20, 20, 20, 20, 20, 20, 20, 20, 20, 20, 20, 20, 20, 20, 20, 20, 20, 20, 20, 20, 20, 20, 20, 20, 20, 20, 20, 20, 20, 20, 20, 20, 20, 20, 20, 20, 20, 20, 20, 20, 20, 20, 20, 20, 20, 20, 20, 20, 20, 20, 20, 20, 20, 20, 20, 20, 20, 20, 20, 20, 20, 20, 20, 20, 20, 20, 20, 20, 20, 20, 20, 20, 20, 20, 20, 20, 20, 20, 20, 20, 20]  InternalRulePriority=Speed  RndMeth=Simplest
  Constant : Constant  Value=uint8(100)
  Constant1 : Constant  Value=uint8(0)
  Enumerated Constant : simulink/Sources/Enumerated Constant  OutDataTypeStr=Enum: VehicleState  Value=VehicleState.ReadyToMove  SampleTime=inf
  Equal : RelationalOperator  Operator===  OutDataTypeStr=boolean  RndMeth=Simplest  InputSameDT=off
  Max : MinMax  Function=max  Inputs=4
  OverMeas : Utilities/OverMeas  sigName='CTRL_WaterPumpDuty_pct'  minimum=0  maximum=100
  Saturation Dynamic : simulink/Discontinuities/Saturation Dynamic  OutMin=[]  OutMax=[]  OutDataTypeStr=Inherit: Same as second input  OutDataType=fixdt(1, 16)  OutScaling=2^-10  DoSatur=off
  Switch : Switch  Criteria=u2 ~= 0  SaturateOnIntegerOverflow=off  InputSameDT=off
  Switch1 : Switch  Criteria=u2 ~= 0  SaturateOnIntegerOverflow=off  InputSameDT=off
  raptor_table_1d : Raptor_lib/Table Lookup/raptor_table_1d  dataName='CTRL_WaterPumpTempToHVDutyCycle'  initValue=[20, 20, 20, 20, 20, 20, 20, 20, 20, 20, 20, 20, 20, 20, 20, 20, 20, 20, 20, 20, 20, 20, 20, 20, 20, 20, 20, 20, 20, 20, 20, 20, 20, 20, 20, 20, 20, 20, 20, 20, 20, 20, 20, 20, 20, 20, 20, 20, 20, 20, 20, 20, 20, 20, 20, 20, 20, 20, 20, 20, 20, 20, 20, 20, 20, 20, 20, 20, 20, 20, 20, 20, 20, 20, 20, 20, 20, 20, 20, 20, 20, 20, 20, 20, 20, 20, 20, 20, 20, 20, 20, 20, 20, 20, 20, 20, 20, 20, 20, 20, 20, 20, 20, 20, 20, 20, 20, 20, 20, 20, 20, 20, 20, 20, 20, 20, 20, 20, 20]  dataType=single  storage=Calibration  initValueX=[0; 1; 2; 3; 4; 5; 6; 7; 8; 9; 10; 11; 12; 13; 14; 15; 16; 17; 18; 19; 20; 21; 22; 23; 24; 25; 26; 27; 28; 29; 30; 31; 32; 33; 34; 35; 36; 37; 38; 39; 40; 41; 42; 43; 44; 45; 46; 47; 48; 49; 50; 51; 52; 53; 54; 55; 56; 57; 58; 59; 60; 61; 62; 63; 64; 65; 66; 67; 68; 69; 70; 71; 72; 73; 74; 75; 76; 77; 78; 79; 80; 81; 82; 83; 84; 85; 86; 87; 88; 89; 90; 91; 92; 93; 94; 95; 96; 97; 98; 99; 100; 101; 102; 103; 104; 105; 106; 107; 108; 109; 110; 111; 112; 113; 114; 115; 116; 117; 118]  dataTypeXY=single  storageXY=Calibration  calVisible=on  showTable=on  calGain=1.0  calOffset=0.0  calMax=Inf  calMin=-Inf  calFormat='-1'  calUnit='pct'  calHelp=''  showBreakpoint=on  dataNameX=[]  calGainX=1.0  calOffsetX=0.0  calMaxX=Inf  calMinX=-Inf  calFormatX='-1'  calUnitX='degC'  calHelpX=''  calAccess=1  calFunction=raptor_xcp_function(gcb)  measureEnable=off  mName=['Data1D_Output']
      settings: SourceProductName=Raptor
  raptor_table_1d1 : Raptor_lib/Table Lookup/raptor_table_1d  dataName='CTRL_WaterPumpTempToLVDutyCycle'  initValue=[20, 20, 20, 20, 20, 20, 20, 20, 20, 20, 20, 20, 20, 20, 20, 20, 20, 20, 20, 20, 20, 20, 20, 20, 20, 20, 20, 20, 20, 20, 20, 20, 20, 20, 20, 20, 20, 20, 20, 20, 20, 20, 20, 20, 20, 20, 20, 20, 20, 20, 20, 20, 20, 20, 20, 20, 20, 20, 20, 20, 20, 20, 20, 20, 20, 20, 20, 20, 20, 20, 20, 20, 20, 20, 20, 20, 20, 20, 20, 20, 20, 20, 20, 20, 20, 20, 20, 20, 20, 20, 20, 20, 20, 20, 20, 20, 20, 20, 20, 20, 20, 20, 20, 20, 20, 20, 20, 20, 20, 20, 20, 20, 20, 20, 20, 20, 20, 20, 20]  dataType=single  storage=Calibration  initValueX=[0; 1; 2; 3; 4; 5; 6; 7; 8; 9; 10; 11; 12; 13; 14; 15; 16; 17; 18; 19; 20; 21; 22; 23; 24; 25; 26; 27; 28; 29; 30; 31; 32; 33; 34; 35; 36; 37; 38; 39; 40; 41; 42; 43; 44; 45; 46; 47; 48; 49; 50; 51; 52; 53; 54; 55; 56; 57; 58; 59; 60; 61; 62; 63; 64; 65; 66; 67; 68; 69; 70; 71; 72; 73; 74; 75; 76; 77; 78; 79; 80; 81; 82; 83; 84; 85; 86; 87; 88; 89; 90; 91; 92; 93; 94; 95; 96; 97; 98; 99; 100; 101; 102; 103; 104; 105; 106; 107; 108; 109; 110; 111; 112; 113; 114; 115; 116; 117; 118]  dataTypeXY=single  storageXY=Calibration  calVisible=on  showTable=on  calGain=1.0  calOffset=0.0  calMax=Inf  calMin=-Inf  calFormat='-1'  calUnit='pct'  calHelp=''  showBreakpoint=on  dataNameX=[]  calGainX=1.0  calOffsetX=0.0  calMaxX=Inf  calMinX=-Inf  calFormatX='-1'  calUnitX='degC'  calHelpX=''  calAccess=1  calFunction=raptor_xcp_function(gcb)  measureEnable=off  mName=['Data1D_Output']
      settings: SourceProductName=Raptor
  raptor_table_1d2 : Raptor_lib/Table Lookup/raptor_table_1d  dataName='CTRL_WaterPumpTempToDutyCycleOverride'  initValue=[20, 20, 20, 20, 20, 20, 20, 20, 20, 20, 20, 20, 20, 20, 20, 20, 20, 20, 20, 20, 20, 20, 20, 20, 20, 20, 20, 20, 20, 20, 20, 20, 20, 20, 20, 20, 20, 20, 20, 20, 20, 20, 20, 20, 20, 20, 20, 20, 20, 20, 20, 20, 20, 20, 20, 20, 20, 20, 20, 20, 20, 20, 20, 20, 20, 20, 20, 20, 20, 20, 20, 20, 20, 20, 20, 20, 20, 20, 20, 20, 20, 20, 20, 20, 20, 20, 20, 20, 20, 20, 20, 20, 20, 20, 20, 20, 20, 20, 20, 20, 20, 20, 20, 20, 20, 20, 20, 20, 20, 20, 20, 20, 20, 20, 20, 20, 20, 20, 20]  dataType=single  storage=Calibration  initValueX=[0; 1; 2; 3; 4; 5; 6; 7; 8; 9; 10; 11; 12; 13; 14; 15; 16; 17; 18; 19; 20; 21; 22; 23; 24; 25; 26; 27; 28; 29; 30; 31; 32; 33; 34; 35; 36; 37; 38; 39; 40; 41; 42; 43; 44; 45; 46; 47; 48; 49; 50; 51; 52; 53; 54; 55; 56; 57; 58; 59; 60; 61; 62; 63; 64; 65; 66; 67; 68; 69; 70; 71; 72; 73; 74; 75; 76; 77; 78; 79; 80; 81; 82; 83; 84; 85; 86; 87; 88; 89; 90; 91; 92; 93; 94; 95; 96; 97; 98; 99; 100; 101; 102; 103; 104; 105; 106; 107; 108; 109; 110; 111; 112; 113; 114; 115; 116; 117; 118]  dataTypeXY=single  storageXY=Calibration  calVisible=on  showTable=on  calGain=1.0  calOffset=0.0  calMax=Inf  calMin=-Inf  calFormat='-1'  calUnit='pct'  calHelp=''  showBreakpoint=on  dataNameX=[]  calGainX=1.0  calOffsetX=0.0  calMaxX=Inf  calMinX=-Inf  calFormatX='-1'  calUnitX='degC'  calHelpX=''  calAccess=1  calFunction=raptor_xcp_function(gcb)  measureEnable=off  mName=['Data1D_Output']
      settings: SourceProductName=Raptor
  DutyCycle : Outport
  wires:
  IN_ModuleCTemp_degC/1 -> Max/4
  CoolSwitch/1 -> Switch1/2
  raptor_table_1d2/1 -> Switch1/1
  Constant/1 -> Saturation Dynamic/1
  Enumerated Constant/1 -> Equal/2
  Constant1/1 -> Saturation Dynamic/3
  Equal/1 -> Switch/2
  OverMeas/1 -> DutyCycle/1  "CTRL_WaterPumpDuty_pct"
  Switch/1 -> Switch1/3
  raptor_table_1d1/1 -> Switch/3
  VehicleState/1 -> Equal/1
  Saturation Dynamic/1 -> OverMeas/1
  IN_ModuleATemp_degC/1 -> Max/2
  Switch1/1 -> Saturation Dynamic/2
  IN_MotorTemp_degC/1 -> Max/1
  raptor_table_1d/1 -> Switch/1
  Max/1 -> raptor_table_1d1/1, raptor_table_1d2/1, raptor_table_1d/1
  IN_ModuleBTemp_degC/1 -> Max/3

== stateflow chart Cooling/CoolButtonLatch ==
  state CoolButtonStop
    en:
    CoolButton = false;
    timer = 0;
  state CoolButtonStart
    en:
    CoolButton = true;
    du:
    timer = timer + dt;
  (default) -> CoolButtonStop
  CoolButtonStop -> CoolButtonStart : [enable == true]
  CoolButtonStart -> CoolButtonStop : [timer > 2000]
  data: enable input; timer local single; dt input; CoolButton output
